simulink library "NeuroModelerLibrary"  (Simulink 10.2)
settings: Solver=ode45  StartTime=0.0  StopTime=10.0  RelTol=1e-3
libraries: $bdroot x672, simulink x5, neural x2
(part 5 of 5)

== system NeuroModelerLibrary/Simple Cells/Simple Cell - Inertial/Synapse ==
  In1 : Inport
  Constant1 : Constant  Value=0
  Constant4 : Constant  Value=DecompositionTC
  Constant5 : Constant  Value=SecretionTC
  Fcn : Fcn  Expr=u*u*ksi
  Gain : Gain  Gain=1/gamma  SaturateOnIntegerOverflow=on  OutDataTypeStr=Inherit: Same as input  ParamDataTypeStr=Inherit: Same as input
  Gain1 : Gain  SaturateOnIntegerOverflow=on  OutDataTypeStr=Inherit: Same as input  ParamDataTypeStr=Inherit: Same as input
  Inertial Link : $bdroot/Support/Inertial Link
  Sum : Sum  Inputs=+-  SaturateOnIntegerOverflow=on
  Switch1 : Switch
  Switch2 : Switch  Threshold=1
  Out1 : Outport  VectorParamsAs1DForOutWhenUnconnected=off
  wires:
  Switch1/1 -> Out1/1
  Gain1/1 -> Inertial Link/1
  Constant1/1 -> Switch1/3
  Gain/1 -> Switch1/1, Switch1/2
  Switch2/1 -> Inertial Link/2
  Constant5/1 -> Switch2/1
  Constant4/1 -> Switch2/3
  Inertial Link/1 -> Sum/1
  Sum/1 -> Gain/1
  In1/1 -> Gain1/1, Switch2/2
  Fcn/1 -> Sum/2

== system NeuroModelerLibrary/Simple Cells/Simple Cell - Inertial/Synapse1 ==
  In1 : Inport
  Constant1 : Constant  Value=0
  Constant4 : Constant  Value=DecompositionTC
  Constant5 : Constant  Value=SecretionTC
  Fcn : Fcn  Expr=u*u*ksi
  Gain : Gain  Gain=1/gamma  SaturateOnIntegerOverflow=on  OutDataTypeStr=Inherit: Same as input  ParamDataTypeStr=Inherit: Same as input
  Gain1 : Gain  SaturateOnIntegerOverflow=on  OutDataTypeStr=Inherit: Same as input  ParamDataTypeStr=Inherit: Same as input
  Inertial Link : $bdroot/Support/Inertial Link
  Sum : Sum  Inputs=+-  SaturateOnIntegerOverflow=on
  Switch1 : Switch
  Switch2 : Switch  Threshold=1
  Out1 : Outport  VectorParamsAs1DForOutWhenUnconnected=off
  wires:
  Switch1/1 -> Out1/1
  Gain1/1 -> Inertial Link/1
  Constant1/1 -> Switch1/3
  Gain/1 -> Switch1/1, Switch1/2
  Switch2/1 -> Inertial Link/2
  Constant5/1 -> Switch2/1
  Constant4/1 -> Switch2/3
  Inertial Link/1 -> Sum/1, Fcn/1
  Sum/1 -> Gain/1
  In1/1 -> Gain1/1, Switch2/2

== system NeuroModelerLibrary/Simple Cells/Simple Cell MembraneCap/Synapse ==
  In1 : Inport
  Constant1 : Constant  Value=0
  Constant4 : Constant  Value=DecompositionTC
  Constant5 : Constant  Value=SecretionTC
  Fcn : Fcn  Expr=u*u*ksi
  Gain : Gain  Gain=1/gamma  SaturateOnIntegerOverflow=on  OutDataTypeStr=Inherit: Same as input  ParamDataTypeStr=Inherit: Same as input
  Gain1 : Gain  SaturateOnIntegerOverflow=on  OutDataTypeStr=Inherit: Same as input  ParamDataTypeStr=Inherit: Same as input
  Inertial Link : $bdroot/Support/Inertial Link  SystemSampleTime=-1  VariantActivationTime=update diagram  Latency=0  AutoFrameSizeCalculation=off
  Sum : Sum  Inputs=+-  SaturateOnIntegerOverflow=on
  Switch1 : Switch
  Switch2 : Switch  Threshold=1
  Out1 : Outport
  wires:
  Fcn/1 -> Sum/2
  In1/1 -> Switch2/2, Gain1/1
  Sum/1 -> Gain/1
  Inertial Link/1 -> Sum/1
  Constant4/1 -> Switch2/3
  Constant5/1 -> Switch2/1
  Switch2/1 -> Inertial Link/2
  Gain/1 -> Switch1/2, Switch1/1
  Constant1/1 -> Switch1/3
  Gain1/1 -> Inertial Link/1
  Switch1/1 -> Out1/1

== system NeuroModelerLibrary/Simple Cells/Simple Cell MembraneCap/Synapse1 ==
  In1 : Inport
  Constant1 : Constant  Value=0
  Constant4 : Constant  Value=DecompositionTC
  Constant5 : Constant  Value=SecretionTC
  Fcn : Fcn  Expr=u*u*ksi
  Gain : Gain  Gain=1/gamma  SaturateOnIntegerOverflow=on  OutDataTypeStr=Inherit: Same as input  ParamDataTypeStr=Inherit: Same as input
  Gain1 : Gain  SaturateOnIntegerOverflow=on  OutDataTypeStr=Inherit: Same as input  ParamDataTypeStr=Inherit: Same as input
  Inertial Link : $bdroot/Support/Inertial Link  SystemSampleTime=-1  VariantActivationTime=update diagram  Latency=0  AutoFrameSizeCalculation=off
  Sum : Sum  Inputs=+-  SaturateOnIntegerOverflow=on
  Switch1 : Switch
  Switch2 : Switch  Threshold=1
  Out1 : Outport
  wires:
  In1/1 -> Switch2/2, Gain1/1
  Sum/1 -> Gain/1
  Inertial Link/1 -> Fcn/1, Sum/1
  Constant4/1 -> Switch2/3
  Constant5/1 -> Switch2/1
  Switch2/1 -> Inertial Link/2
  Gain/1 -> Switch1/2, Switch1/1
  Constant1/1 -> Switch1/3
  Gain1/1 -> Inertial Link/1
  Switch1/1 -> Out1/1

== system NeuroModelerLibrary/Simple Cells/Simple Cell MembraneCap[2]/Synapse ==
  In1 : Inport
  Constant1 : Constant  Value=0
  Constant4 : Constant  Value=DecompositionTC
  Constant5 : Constant  Value=SecretionTC
  Fcn : Fcn  Expr=u*u*ksi
  Gain : Gain  Gain=1/gamma  SaturateOnIntegerOverflow=on  OutDataTypeStr=Inherit: Same as input  ParamDataTypeStr=Inherit: Same as input
  Gain1 : Gain  SaturateOnIntegerOverflow=on  OutDataTypeStr=Inherit: Same as input  ParamDataTypeStr=Inherit: Same as input
  Inertial Link : $bdroot/Support/Inertial Link  SystemSampleTime=-1  VariantActivationTime=update diagram  Latency=0  AutoFrameSizeCalculation=off
  Sum : Sum  Inputs=+-  SaturateOnIntegerOverflow=on
  Switch1 : Switch
  Switch2 : Switch  Threshold=1
  Out1 : Outport
  wires:
  Fcn/1 -> Sum/2
  In1/1 -> Switch2/2, Gain1/1
  Sum/1 -> Gain/1
  Inertial Link/1 -> Sum/1
  Constant4/1 -> Switch2/3
  Constant5/1 -> Switch2/1
  Switch2/1 -> Inertial Link/2
  Gain/1 -> Switch1/2, Switch1/1
  Constant1/1 -> Switch1/3
  Gain1/1 -> Inertial Link/1
  Switch1/1 -> Out1/1

== system NeuroModelerLibrary/Simple Cells/Simple Cell MembraneCap[2]/Synapse1 ==
  In1 : Inport
  Constant1 : Constant  Value=0
  Constant4 : Constant  Value=DecompositionTC
  Constant5 : Constant  Value=SecretionTC
  Fcn : Fcn  Expr=u*u*ksi
  Gain : Gain  Gain=1/gamma  SaturateOnIntegerOverflow=on  OutDataTypeStr=Inherit: Same as input  ParamDataTypeStr=Inherit: Same as input
  Gain1 : Gain  SaturateOnIntegerOverflow=on  OutDataTypeStr=Inherit: Same as input  ParamDataTypeStr=Inherit: Same as input
  Inertial Link : $bdroot/Support/Inertial Link  SystemSampleTime=-1  VariantActivationTime=update diagram  Latency=0  AutoFrameSizeCalculation=off
  Sum : Sum  Inputs=+-  SaturateOnIntegerOverflow=on
  Switch1 : Switch
  Switch2 : Switch  Threshold=1
  Out1 : Outport
  wires:
  In1/1 -> Switch2/2, Gain1/1
  Sum/1 -> Gain/1
  Inertial Link/1 -> Fcn/1, Sum/1
  Constant4/1 -> Switch2/3
  Constant5/1 -> Switch2/1
  Switch2/1 -> Inertial Link/2
  Gain/1 -> Switch1/2, Switch1/1
  Constant1/1 -> Switch1/3
  Gain1/1 -> Inertial Link/1
  Switch1/1 -> Out1/1

== system NeuroModelerLibrary/Sized Cells/Cell IaF 1x4/IaF LTZone6 ==
  Potential : Inport
  Constant2 : Constant
  Constant6 : Constant  Value=0
  S1 : Switch  Threshold=V_th  SaturateOnIntegerOverflow=on  InputSameDT=on
  Out : Outport
  Out Potential : Outport  Port=2
  wires:
  Constant2/1 -> S1/1
  Constant6/1 -> S1/3
  Potential/1 -> Out Potential/1, S1/2
  S1/1 -> Out/1

== system NeuroModelerLibrary/Sized Cells/Cell IaF 1x4/IaF Membrane Segment18 ==
  Synapses : Inport
  Resting Potential : Inport  Port=2
  Reset Signal : Inport  Port=3
  Constant1 : Constant  Value=V_reset
  Constant10 : Constant  Value=tau_m
  Constant12 : Constant  Value=I_const
  Gain3 : Gain  Gain=tau_m/Cm
  Inertial Link With Reset1 : $bdroot/Support/Inertial Link With Reset  SystemSampleTime=-1  VariantActivationTime=update diagram  Latency=0  AutoFrameSizeCalculation=off
  Sum1 : Sum
  Sum3 : Sum
  Out1 : Outport
  wires:
  Resting Potential/1 -> Sum3/2
  Constant10/1 -> Inertial Link With Reset1/2
  Synapses/1 -> Sum1/1
  Sum1/1 -> Gain3/1
  Constant12/1 -> Sum1/2
  Sum3/1 -> Inertial Link With Reset1/1  "Value"
  Inertial Link With Reset1/1 -> Out1/1
  Constant1/1 -> Inertial Link With Reset1/3
  Gain3/1 -> Sum3/1  "Input"
  Reset Signal/1 -> Inertial Link With Reset1/4

== system NeuroModelerLibrary/Sized Cells/Cell IaF 1x4/IaF Membrane Segment19 ==
  Synapses : Inport
  Resting Potential : Inport  Port=2
  Reset Signal : Inport  Port=3
  Constant1 : Constant  Value=V_reset
  Constant10 : Constant  Value=tau_m
  Constant12 : Constant  Value=I_const
  Gain3 : Gain  Gain=tau_m/Cm
  Inertial Link With Reset1 : $bdroot/Support/Inertial Link With Reset  SystemSampleTime=-1  VariantActivationTime=update diagram  Latency=0  AutoFrameSizeCalculation=off
  Sum1 : Sum
  Sum3 : Sum
  Out1 : Outport
  wires:
  Resting Potential/1 -> Sum3/2
  Constant10/1 -> Inertial Link With Reset1/2
  Synapses/1 -> Sum1/1
  Sum1/1 -> Gain3/1
  Constant12/1 -> Sum1/2
  Sum3/1 -> Inertial Link With Reset1/1  "Value"
  Inertial Link With Reset1/1 -> Out1/1
  Constant1/1 -> Inertial Link With Reset1/3
  Gain3/1 -> Sum3/1  "Input"
  Reset Signal/1 -> Inertial Link With Reset1/4

== system NeuroModelerLibrary/Sized Cells/Cell IaF 1x4/IaF Membrane Segment20 ==
  Synapses : Inport
  Resting Potential : Inport  Port=2
  Reset Signal : Inport  Port=3
  Constant1 : Constant  Value=V_reset
  Constant10 : Constant  Value=tau_m
  Constant12 : Constant  Value=I_const
  Gain3 : Gain  Gain=tau_m/Cm
  Inertial Link With Reset1 : $bdroot/Support/Inertial Link With Reset  SystemSampleTime=-1  VariantActivationTime=update diagram  Latency=0  AutoFrameSizeCalculation=off
  Sum1 : Sum
  Sum3 : Sum
  Out1 : Outport
  wires:
  Resting Potential/1 -> Sum3/2
  Constant10/1 -> Inertial Link With Reset1/2
  Synapses/1 -> Sum1/1
  Sum1/1 -> Gain3/1
  Constant12/1 -> Sum1/2
  Sum3/1 -> Inertial Link With Reset1/1  "Value"
  Inertial Link With Reset1/1 -> Out1/1
  Constant1/1 -> Inertial Link With Reset1/3
  Gain3/1 -> Sum3/1  "Input"
  Reset Signal/1 -> Inertial Link With Reset1/4

== system NeuroModelerLibrary/Sized Cells/Cell IaF 1x4/IaF Membrane Segment21 ==
  Synapses : Inport
  Resting Potential : Inport  Port=2
  Reset Signal : Inport  Port=3
  Constant1 : Constant  Value=V_reset
  Constant10 : Constant  Value=tau_m
  Constant12 : Constant  Value=I_const
  Gain3 : Gain  Gain=tau_m/Cm
  Inertial Link With Reset1 : $bdroot/Support/Inertial Link With Reset  SystemSampleTime=-1  VariantActivationTime=update diagram  Latency=0  AutoFrameSizeCalculation=off
  Sum1 : Sum
  Sum3 : Sum
  Out1 : Outport
  wires:
  Resting Potential/1 -> Sum3/2
  Constant10/1 -> Inertial Link With Reset1/2
  Synapses/1 -> Sum1/1
  Sum1/1 -> Gain3/1
  Constant12/1 -> Sum1/2
  Sum3/1 -> Inertial Link With Reset1/1  "Value"
  Inertial Link With Reset1/1 -> Out1/1
  Constant1/1 -> Inertial Link With Reset1/3
  Gain3/1 -> Sum3/1  "Input"
  Reset Signal/1 -> Inertial Link With Reset1/4

== system NeuroModelerLibrary/Sized Cells/Cell IaF 1x4-Syn4/IaF LTZone1 ==
  Potential : Inport
  Constant2 : Constant
  Constant6 : Constant  Value=0
  S1 : Switch  Threshold=V_th  SaturateOnIntegerOverflow=on  InputSameDT=on
  Out : Outport
  Out Potential : Outport  Port=2
  wires:
  Constant2/1 -> S1/1
  Constant6/1 -> S1/3
  Potential/1 -> Out Potential/1, S1/2
  S1/1 -> Out/1

== system NeuroModelerLibrary/Sized Cells/Cell IaF 1x4-Syn4/IaF Membrane Segment1 ==
  Synapses : Inport
  Resting Potential : Inport  Port=2
  Reset Signal : Inport  Port=3
  Constant1 : Constant  Value=V_reset
  Constant10 : Constant  Value=tau_m
  Constant12 : Constant  Value=I_const
  Gain3 : Gain  Gain=tau_m/Cm
  Inertial Link With Reset1 : $bdroot/Support/Inertial Link With Reset  SystemSampleTime=-1  VariantActivationTime=update diagram  Latency=0  AutoFrameSizeCalculation=off
  Sum1 : Sum
  Sum3 : Sum
  Out1 : Outport
  wires:
  Resting Potential/1 -> Sum3/2
  Constant10/1 -> Inertial Link With Reset1/2
  Synapses/1 -> Sum1/1
  Sum1/1 -> Gain3/1
  Constant12/1 -> Sum1/2
  Sum3/1 -> Inertial Link With Reset1/1  "Value"
  Inertial Link With Reset1/1 -> Out1/1
  Constant1/1 -> Inertial Link With Reset1/3
  Gain3/1 -> Sum3/1  "Input"
  Reset Signal/1 -> Inertial Link With Reset1/4

== system NeuroModelerLibrary/Sized Cells/Cell IaF 1x4-Syn4/IaF Membrane Segment2 ==
  Synapses : Inport
  Resting Potential : Inport  Port=2
  Reset Signal : Inport  Port=3
  Constant1 : Constant  Value=V_reset
  Constant10 : Constant  Value=tau_m
  Constant12 : Constant  Value=I_const
  Gain3 : Gain  Gain=tau_m/Cm
  Inertial Link With Reset1 : $bdroot/Support/Inertial Link With Reset  SystemSampleTime=-1  VariantActivationTime=update diagram  Latency=0  AutoFrameSizeCalculation=off
  Sum1 : Sum
  Sum3 : Sum
  Out1 : Outport
  wires:
  Resting Potential/1 -> Sum3/2
  Constant10/1 -> Inertial Link With Reset1/2
  Synapses/1 -> Sum1/1
  Sum1/1 -> Gain3/1
  Constant12/1 -> Sum1/2
  Sum3/1 -> Inertial Link With Reset1/1  "Value"
  Inertial Link With Reset1/1 -> Out1/1
  Constant1/1 -> Inertial Link With Reset1/3
  Gain3/1 -> Sum3/1  "Input"
  Reset Signal/1 -> Inertial Link With Reset1/4

== system NeuroModelerLibrary/Sized Cells/Cell IaF 1x4-Syn4/IaF Membrane Segment3 ==
  Synapses : Inport
  Resting Potential : Inport  Port=2
  Reset Signal : Inport  Port=3
  Constant1 : Constant  Value=V_reset
  Constant10 : Constant  Value=tau_m
  Constant12 : Constant  Value=I_const
  Gain3 : Gain  Gain=tau_m/Cm
  Inertial Link With Reset1 : $bdroot/Support/Inertial Link With Reset  SystemSampleTime=-1  VariantActivationTime=update diagram  Latency=0  AutoFrameSizeCalculation=off
  Sum1 : Sum
  Sum3 : Sum
  Out1 : Outport
  wires:
  Resting Potential/1 -> Sum3/2
  Constant10/1 -> Inertial Link With Reset1/2
  Synapses/1 -> Sum1/1
  Sum1/1 -> Gain3/1
  Constant12/1 -> Sum1/2
  Sum3/1 -> Inertial Link With Reset1/1  "Value"
  Inertial Link With Reset1/1 -> Out1/1
  Constant1/1 -> Inertial Link With Reset1/3
  Gain3/1 -> Sum3/1  "Input"
  Reset Signal/1 -> Inertial Link With Reset1/4

== system NeuroModelerLibrary/Sized Cells/Cell IaF 1x4-Syn4/IaF Membrane Segment4 ==
  Synapses : Inport
  Resting Potential : Inport  Port=2
  Reset Signal : Inport  Port=3
  Constant1 : Constant  Value=V_reset
  Constant10 : Constant  Value=tau_m
  Constant12 : Constant  Value=I_const
  Gain3 : Gain  Gain=tau_m/Cm
  Inertial Link With Reset1 : $bdroot/Support/Inertial Link With Reset  SystemSampleTime=-1  VariantActivationTime=update diagram  Latency=0  AutoFrameSizeCalculation=off
  Sum1 : Sum
  Sum3 : Sum
  Out1 : Outport
  wires:
  Resting Potential/1 -> Sum3/2
  Constant10/1 -> Inertial Link With Reset1/2
  Synapses/1 -> Sum1/1
  Sum1/1 -> Gain3/1
  Constant12/1 -> Sum1/2
  Sum3/1 -> Inertial Link With Reset1/1  "Value"
  Inertial Link With Reset1/1 -> Out1/1
  Constant1/1 -> Inertial Link With Reset1/3
  Gain3/1 -> Sum3/1  "Input"
  Reset Signal/1 -> Inertial Link With Reset1/4

== system NeuroModelerLibrary/Sized Cells/Cell IaF 2x4/IaF LTZone7 ==
  Potential : Inport
  Constant2 : Constant
  Constant6 : Constant  Value=0
  S1 : Switch  Threshold=V_th  SaturateOnIntegerOverflow=on  InputSameDT=on
  Out : Outport
  Out Potential : Outport  Port=2
  wires:
  Constant2/1 -> S1/1
  Constant6/1 -> S1/3
  Potential/1 -> Out Potential/1, S1/2
  S1/1 -> Out/1

== system NeuroModelerLibrary/Sized Cells/Cell IaF 2x4/IaF Membrane Segment22 ==
  Synapses : Inport
  Resting Potential : Inport  Port=2
  Reset Signal : Inport  Port=3
  Constant1 : Constant  Value=V_reset
  Constant10 : Constant  Value=tau_m
  Constant12 : Constant  Value=I_const
  Gain3 : Gain  Gain=tau_m/Cm
  Inertial Link With Reset1 : $bdroot/Support/Inertial Link With Reset  SystemSampleTime=-1  VariantActivationTime=update diagram  Latency=0  AutoFrameSizeCalculation=off
  Sum1 : Sum
  Sum3 : Sum
  Out1 : Outport
  wires:
  Resting Potential/1 -> Sum3/2
  Constant10/1 -> Inertial Link With Reset1/2
  Synapses/1 -> Sum1/1
  Sum1/1 -> Gain3/1
  Constant12/1 -> Sum1/2
  Sum3/1 -> Inertial Link With Reset1/1  "Value"
  Inertial Link With Reset1/1 -> Out1/1
  Constant1/1 -> Inertial Link With Reset1/3
  Gain3/1 -> Sum3/1  "Input"
  Reset Signal/1 -> Inertial Link With Reset1/4

== system NeuroModelerLibrary/Sized Cells/Cell IaF 2x4/IaF Membrane Segment23 ==
  Synapses : Inport
  Resting Potential : Inport  Port=2
  Reset Signal : Inport  Port=3
  Constant1 : Constant  Value=V_reset
  Constant10 : Constant  Value=tau_m
  Constant12 : Constant  Value=I_const
  Gain3 : Gain  Gain=tau_m/Cm
  Inertial Link With Reset1 : $bdroot/Support/Inertial Link With Reset  SystemSampleTime=-1  VariantActivationTime=update diagram  Latency=0  AutoFrameSizeCalculation=off
  Sum1 : Sum
  Sum3 : Sum
  Out1 : Outport
  wires:
  Resting Potential/1 -> Sum3/2
  Constant10/1 -> Inertial Link With Reset1/2
  Synapses/1 -> Sum1/1
  Sum1/1 -> Gain3/1
  Constant12/1 -> Sum1/2
  Sum3/1 -> Inertial Link With Reset1/1  "Value"
  Inertial Link With Reset1/1 -> Out1/1
  Constant1/1 -> Inertial Link With Reset1/3
  Gain3/1 -> Sum3/1  "Input"
  Reset Signal/1 -> Inertial Link With Reset1/4

== system NeuroModelerLibrary/Sized Cells/Cell IaF 2x4/IaF Membrane Segment24 ==
  Synapses : Inport
  Resting Potential : Inport  Port=2
  Reset Signal : Inport  Port=3
  Constant1 : Constant  Value=V_reset
  Constant10 : Constant  Value=tau_m
  Constant12 : Constant  Value=I_const
  Gain3 : Gain  Gain=tau_m/Cm
  Inertial Link With Reset1 : $bdroot/Support/Inertial Link With Reset  SystemSampleTime=-1  VariantActivationTime=update diagram  Latency=0  AutoFrameSizeCalculation=off
  Sum1 : Sum
  Sum3 : Sum
  Out1 : Outport
  wires:
  Resting Potential/1 -> Sum3/2
  Constant10/1 -> Inertial Link With Reset1/2
  Synapses/1 -> Sum1/1
  Sum1/1 -> Gain3/1
  Constant12/1 -> Sum1/2
  Sum3/1 -> Inertial Link With Reset1/1  "Value"
  Inertial Link With Reset1/1 -> Out1/1
  Constant1/1 -> Inertial Link With Reset1/3
  Gain3/1 -> Sum3/1  "Input"
  Reset Signal/1 -> Inertial Link With Reset1/4

== system NeuroModelerLibrary/Sized Cells/Cell IaF 2x4/IaF Membrane Segment25 ==
  Synapses : Inport
  Resting Potential : Inport  Port=2
  Reset Signal : Inport  Port=3
  Constant1 : Constant  Value=V_reset
  Constant10 : Constant  Value=tau_m
  Constant12 : Constant  Value=I_const
  Gain3 : Gain  Gain=tau_m/Cm
  Inertial Link With Reset1 : $bdroot/Support/Inertial Link With Reset  SystemSampleTime=-1  VariantActivationTime=update diagram  Latency=0  AutoFrameSizeCalculation=off
  Sum1 : Sum
  Sum3 : Sum
  Out1 : Outport
  wires:
  Resting Potential/1 -> Sum3/2
  Constant10/1 -> Inertial Link With Reset1/2
  Synapses/1 -> Sum1/1
  Sum1/1 -> Gain3/1
  Constant12/1 -> Sum1/2
  Sum3/1 -> Inertial Link With Reset1/1  "Value"
  Inertial Link With Reset1/1 -> Out1/1
  Constant1/1 -> Inertial Link With Reset1/3
  Gain3/1 -> Sum3/1  "Input"
  Reset Signal/1 -> Inertial Link With Reset1/4

== system NeuroModelerLibrary/Sized Cells/Cell IaF 2x4/IaF Membrane Segment26 ==
  Synapses : Inport
  Resting Potential : Inport  Port=2
  Reset Signal : Inport  Port=3
  Constant1 : Constant  Value=V_reset
  Constant10 : Constant  Value=tau_m
  Constant12 : Constant  Value=I_const
  Gain3 : Gain  Gain=tau_m/Cm
  Inertial Link With Reset1 : $bdroot/Support/Inertial Link With Reset  SystemSampleTime=-1  VariantActivationTime=update diagram  Latency=0  AutoFrameSizeCalculation=off
  Sum1 : Sum
  Sum3 : Sum
  Out1 : Outport
  wires:
  Resting Potential/1 -> Sum3/2
  Constant10/1 -> Inertial Link With Reset1/2
  Synapses/1 -> Sum1/1
  Sum1/1 -> Gain3/1
  Constant12/1 -> Sum1/2
  Sum3/1 -> Inertial Link With Reset1/1  "Value"
  Inertial Link With Reset1/1 -> Out1/1
  Constant1/1 -> Inertial Link With Reset1/3
  Gain3/1 -> Sum3/1  "Input"
  Reset Signal/1 -> Inertial Link With Reset1/4

== system NeuroModelerLibrary/Sized Cells/Cell IaF 3x4/IaF LTZone8 ==
  Potential : Inport
  Constant2 : Constant
  Constant6 : Constant  Value=0
  S1 : Switch  Threshold=V_th  SaturateOnIntegerOverflow=on  InputSameDT=on
  Out : Outport
  Out Potential : Outport  Port=2
  wires:
  Constant2/1 -> S1/1
  Constant6/1 -> S1/3
  Potential/1 -> Out Potential/1, S1/2
  S1/1 -> Out/1

== system NeuroModelerLibrary/Sized Cells/Cell IaF 3x4/IaF Membrane Segment27 ==
  Synapses : Inport
  Resting Potential : Inport  Port=2
  Reset Signal : Inport  Port=3
  Constant1 : Constant  Value=V_reset
  Constant10 : Constant  Value=tau_m
  Constant12 : Constant  Value=I_const
  Gain3 : Gain  Gain=tau_m/Cm
  Inertial Link With Reset1 : $bdroot/Support/Inertial Link With Reset  SystemSampleTime=-1  VariantActivationTime=update diagram  Latency=0  AutoFrameSizeCalculation=off
  Sum1 : Sum
  Sum3 : Sum
  Out1 : Outport
  wires:
  Resting Potential/1 -> Sum3/2
  Constant10/1 -> Inertial Link With Reset1/2
  Synapses/1 -> Sum1/1
  Sum1/1 -> Gain3/1
  Constant12/1 -> Sum1/2
  Sum3/1 -> Inertial Link With Reset1/1  "Value"
  Inertial Link With Reset1/1 -> Out1/1
  Constant1/1 -> Inertial Link With Reset1/3
  Gain3/1 -> Sum3/1  "Input"
  Reset Signal/1 -> Inertial Link With Reset1/4

== system NeuroModelerLibrary/Sized Cells/Cell IaF 3x4/IaF Membrane Segment28 ==
  Synapses : Inport
  Resting Potential : Inport  Port=2
  Reset Signal : Inport  Port=3
  Constant1 : Constant  Value=V_reset
  Constant10 : Constant  Value=tau_m
  Constant12 : Constant  Value=I_const
  Gain3 : Gain  Gain=tau_m/Cm
  Inertial Link With Reset1 : $bdroot/Support/Inertial Link With Reset  SystemSampleTime=-1  VariantActivationTime=update diagram  Latency=0  AutoFrameSizeCalculation=off
  Sum1 : Sum
  Sum3 : Sum
  Out1 : Outport
  wires:
  Resting Potential/1 -> Sum3/2
  Constant10/1 -> Inertial Link With Reset1/2
  Synapses/1 -> Sum1/1
  Sum1/1 -> Gain3/1
  Constant12/1 -> Sum1/2
  Sum3/1 -> Inertial Link With Reset1/1  "Value"
  Inertial Link With Reset1/1 -> Out1/1
  Constant1/1 -> Inertial Link With Reset1/3
  Gain3/1 -> Sum3/1  "Input"
  Reset Signal/1 -> Inertial Link With Reset1/4

== system NeuroModelerLibrary/Sized Cells/Cell IaF 3x4/IaF Membrane Segment29 ==
  Synapses : Inport
  Resting Potential : Inport  Port=2
  Reset Signal : Inport  Port=3
  Constant1 : Constant  Value=V_reset
  Constant10 : Constant  Value=tau_m
  Constant12 : Constant  Value=I_const
  Gain3 : Gain  Gain=tau_m/Cm
  Inertial Link With Reset1 : $bdroot/Support/Inertial Link With Reset  SystemSampleTime=-1  VariantActivationTime=update diagram  Latency=0  AutoFrameSizeCalculation=off
  Sum1 : Sum
  Sum3 : Sum
  Out1 : Outport
  wires:
  Resting Potential/1 -> Sum3/2
  Constant10/1 -> Inertial Link With Reset1/2
  Synapses/1 -> Sum1/1
  Sum1/1 -> Gain3/1
  Constant12/1 -> Sum1/2
  Sum3/1 -> Inertial Link With Reset1/1  "Value"
  Inertial Link With Reset1/1 -> Out1/1
  Constant1/1 -> Inertial Link With Reset1/3
  Gain3/1 -> Sum3/1  "Input"
  Reset Signal/1 -> Inertial Link With Reset1/4

== system NeuroModelerLibrary/Sized Cells/Cell IaF 3x4/IaF Membrane Segment30 ==
  Synapses : Inport
  Resting Potential : Inport  Port=2
  Reset Signal : Inport  Port=3
  Constant1 : Constant  Value=V_reset
  Constant10 : Constant  Value=tau_m
  Constant12 : Constant  Value=I_const
  Gain3 : Gain  Gain=tau_m/Cm
  Inertial Link With Reset1 : $bdroot/Support/Inertial Link With Reset  SystemSampleTime=-1  VariantActivationTime=update diagram  Latency=0  AutoFrameSizeCalculation=off
  Sum1 : Sum
  Sum3 : Sum
  Out1 : Outport
  wires:
  Resting Potential/1 -> Sum3/2
  Constant10/1 -> Inertial Link With Reset1/2
  Synapses/1 -> Sum1/1
  Sum1/1 -> Gain3/1
  Constant12/1 -> Sum1/2
  Sum3/1 -> Inertial Link With Reset1/1  "Value"
  Inertial Link With Reset1/1 -> Out1/1
  Constant1/1 -> Inertial Link With Reset1/3
  Gain3/1 -> Sum3/1  "Input"
  Reset Signal/1 -> Inertial Link With Reset1/4

== system NeuroModelerLibrary/Sized Cells/Cell IaF 3x4/IaF Membrane Segment31 ==
  Synapses : Inport
  Resting Potential : Inport  Port=2
  Reset Signal : Inport  Port=3
  Constant1 : Constant  Value=V_reset
  Constant10 : Constant  Value=tau_m
  Constant12 : Constant  Value=I_const
  Gain3 : Gain  Gain=tau_m/Cm
  Inertial Link With Reset1 : $bdroot/Support/Inertial Link With Reset  SystemSampleTime=-1  VariantActivationTime=update diagram  Latency=0  AutoFrameSizeCalculation=off
  Sum1 : Sum
  Sum3 : Sum
  Out1 : Outport
  wires:
  Resting Potential/1 -> Sum3/2
  Constant10/1 -> Inertial Link With Reset1/2
  Synapses/1 -> Sum1/1
  Sum1/1 -> Gain3/1
  Constant12/1 -> Sum1/2
  Sum3/1 -> Inertial Link With Reset1/1  "Value"
  Inertial Link With Reset1/1 -> Out1/1
  Constant1/1 -> Inertial Link With Reset1/3
  Gain3/1 -> Sum3/1  "Input"
  Reset Signal/1 -> Inertial Link With Reset1/4

== system NeuroModelerLibrary/Sized Cells/Cell IaF 3x4/IaF Membrane Segment32 ==
  Synapses : Inport
  Resting Potential : Inport  Port=2
  Reset Signal : Inport  Port=3
  Constant1 : Constant  Value=V_reset
  Constant10 : Constant  Value=tau_m
  Constant12 : Constant  Value=I_const
  Gain3 : Gain  Gain=tau_m/Cm
  Inertial Link With Reset1 : $bdroot/Support/Inertial Link With Reset  SystemSampleTime=-1  VariantActivationTime=update diagram  Latency=0  AutoFrameSizeCalculation=off
  Sum1 : Sum
  Sum3 : Sum
  Out1 : Outport
  wires:
  Resting Potential/1 -> Sum3/2
  Constant10/1 -> Inertial Link With Reset1/2
  Synapses/1 -> Sum1/1
  Sum1/1 -> Gain3/1
  Constant12/1 -> Sum1/2
  Sum3/1 -> Inertial Link With Reset1/1  "Value"
  Inertial Link With Reset1/1 -> Out1/1
  Constant1/1 -> Inertial Link With Reset1/3
  Gain3/1 -> Sum3/1  "Input"
  Reset Signal/1 -> Inertial Link With Reset1/4

== system NeuroModelerLibrary/Sized Cells/Cell IaF 4x4/IaF LTZone9 ==
  Potential : Inport
  Constant2 : Constant
  Constant6 : Constant  Value=0
  S1 : Switch  Threshold=V_th  SaturateOnIntegerOverflow=on  InputSameDT=on
  Out : Outport
  Out Potential : Outport  Port=2
  wires:
  Constant2/1 -> S1/1
  Constant6/1 -> S1/3
  Potential/1 -> Out Potential/1, S1/2
  S1/1 -> Out/1

== system NeuroModelerLibrary/Sized Cells/Cell IaF 4x4/IaF Membrane Segment33 ==
  Synapses : Inport
  Resting Potential : Inport  Port=2
  Reset Signal : Inport  Port=3
  Constant1 : Constant  Value=V_reset
  Constant10 : Constant  Value=tau_m
  Constant12 : Constant  Value=I_const
  Gain3 : Gain  Gain=tau_m/Cm
  Inertial Link With Reset1 : $bdroot/Support/Inertial Link With Reset  SystemSampleTime=-1  VariantActivationTime=update diagram  Latency=0  AutoFrameSizeCalculation=off
  Sum1 : Sum
  Sum3 : Sum
  Out1 : Outport
  wires:
  Resting Potential/1 -> Sum3/2
  Constant10/1 -> Inertial Link With Reset1/2
  Synapses/1 -> Sum1/1
  Sum1/1 -> Gain3/1
  Constant12/1 -> Sum1/2
  Sum3/1 -> Inertial Link With Reset1/1  "Value"
  Inertial Link With Reset1/1 -> Out1/1
  Constant1/1 -> Inertial Link With Reset1/3
  Gain3/1 -> Sum3/1  "Input"
  Reset Signal/1 -> Inertial Link With Reset1/4

== system NeuroModelerLibrary/Sized Cells/Cell IaF 4x4/IaF Membrane Segment34 ==
  Synapses : Inport
  Resting Potential : Inport  Port=2
  Reset Signal : Inport  Port=3
  Constant1 : Constant  Value=V_reset
  Constant10 : Constant  Value=tau_m
  Constant12 : Constant  Value=I_const
  Gain3 : Gain  Gain=tau_m/Cm
  Inertial Link With Reset1 : $bdroot/Support/Inertial Link With Reset  SystemSampleTime=-1  VariantActivationTime=update diagram  Latency=0  AutoFrameSizeCalculation=off
  Sum1 : Sum
  Sum3 : Sum
  Out1 : Outport
  wires:
  Resting Potential/1 -> Sum3/2
  Constant10/1 -> Inertial Link With Reset1/2
  Synapses/1 -> Sum1/1
  Sum1/1 -> Gain3/1
  Constant12/1 -> Sum1/2
  Sum3/1 -> Inertial Link With Reset1/1  "Value"
  Inertial Link With Reset1/1 -> Out1/1
  Constant1/1 -> Inertial Link With Reset1/3
  Gain3/1 -> Sum3/1  "Input"
  Reset Signal/1 -> Inertial Link With Reset1/4

== system NeuroModelerLibrary/Sized Cells/Cell IaF 4x4/IaF Membrane Segment35 ==
  Synapses : Inport
  Resting Potential : Inport  Port=2
  Reset Signal : Inport  Port=3
  Constant1 : Constant  Value=V_reset
  Constant10 : Constant  Value=tau_m
  Constant12 : Constant  Value=I_const
  Gain3 : Gain  Gain=tau_m/Cm
  Inertial Link With Reset1 : $bdroot/Support/Inertial Link With Reset  SystemSampleTime=-1  VariantActivationTime=update diagram  Latency=0  AutoFrameSizeCalculation=off
  Sum1 : Sum
  Sum3 : Sum
  Out1 : Outport
  wires:
  Resting Potential/1 -> Sum3/2
  Constant10/1 -> Inertial Link With Reset1/2
  Synapses/1 -> Sum1/1
  Sum1/1 -> Gain3/1
  Constant12/1 -> Sum1/2
  Sum3/1 -> Inertial Link With Reset1/1  "Value"
  Inertial Link With Reset1/1 -> Out1/1
  Constant1/1 -> Inertial Link With Reset1/3
  Gain3/1 -> Sum3/1  "Input"
  Reset Signal/1 -> Inertial Link With Reset1/4

== system NeuroModelerLibrary/Sized Cells/Cell IaF 4x4/IaF Membrane Segment36 ==
  Synapses : Inport
  Resting Potential : Inport  Port=2
  Reset Signal : Inport  Port=3
  Constant1 : Constant  Value=V_reset
  Constant10 : Constant  Value=tau_m
  Constant12 : Constant  Value=I_const
  Gain3 : Gain  Gain=tau_m/Cm
  Inertial Link With Reset1 : $bdroot/Support/Inertial Link With Reset  SystemSampleTime=-1  VariantActivationTime=update diagram  Latency=0  AutoFrameSizeCalculation=off
  Sum1 : Sum
  Sum3 : Sum
  Out1 : Outport
  wires:
  Resting Potential/1 -> Sum3/2
  Constant10/1 -> Inertial Link With Reset1/2
  Synapses/1 -> Sum1/1
  Sum1/1 -> Gain3/1
  Constant12/1 -> Sum1/2
  Sum3/1 -> Inertial Link With Reset1/1  "Value"
  Inertial Link With Reset1/1 -> Out1/1
  Constant1/1 -> Inertial Link With Reset1/3
  Gain3/1 -> Sum3/1  "Input"
  Reset Signal/1 -> Inertial Link With Reset1/4

== system NeuroModelerLibrary/Sized Cells/Cell IaF 4x4/IaF Membrane Segment37 ==
  Synapses : Inport
  Resting Potential : Inport  Port=2
  Reset Signal : Inport  Port=3
  Constant1 : Constant  Value=V_reset
  Constant10 : Constant  Value=tau_m
  Constant12 : Constant  Value=I_const
  Gain3 : Gain  Gain=tau_m/Cm
  Inertial Link With Reset1 : $bdroot/Support/Inertial Link With Reset  SystemSampleTime=-1  VariantActivationTime=update diagram  Latency=0  AutoFrameSizeCalculation=off
  Sum1 : Sum
  Sum3 : Sum
  Out1 : Outport
  wires:
  Resting Potential/1 -> Sum3/2
  Constant10/1 -> Inertial Link With Reset1/2
  Synapses/1 -> Sum1/1
  Sum1/1 -> Gain3/1
  Constant12/1 -> Sum1/2
  Sum3/1 -> Inertial Link With Reset1/1  "Value"
  Inertial Link With Reset1/1 -> Out1/1
  Constant1/1 -> Inertial Link With Reset1/3
  Gain3/1 -> Sum3/1  "Input"
  Reset Signal/1 -> Inertial Link With Reset1/4

== system NeuroModelerLibrary/Sized Cells/Cell IaF 4x4/IaF Membrane Segment38 ==
  Synapses : Inport
  Resting Potential : Inport  Port=2
  Reset Signal : Inport  Port=3
  Constant1 : Constant  Value=V_reset
  Constant10 : Constant  Value=tau_m
  Constant12 : Constant  Value=I_const
  Gain3 : Gain  Gain=tau_m/Cm
  Inertial Link With Reset1 : $bdroot/Support/Inertial Link With Reset  SystemSampleTime=-1  VariantActivationTime=update diagram  Latency=0  AutoFrameSizeCalculation=off
  Sum1 : Sum
  Sum3 : Sum
  Out1 : Outport
  wires:
  Resting Potential/1 -> Sum3/2
  Constant10/1 -> Inertial Link With Reset1/2
  Synapses/1 -> Sum1/1
  Sum1/1 -> Gain3/1
  Constant12/1 -> Sum1/2
  Sum3/1 -> Inertial Link With Reset1/1  "Value"
  Inertial Link With Reset1/1 -> Out1/1
  Constant1/1 -> Inertial Link With Reset1/3
  Gain3/1 -> Sum3/1  "Input"
  Reset Signal/1 -> Inertial Link With Reset1/4

== system NeuroModelerLibrary/Sized Cells/Cell IaF 4x4/IaF Membrane Segment39 ==
  Synapses : Inport
  Resting Potential : Inport  Port=2
  Reset Signal : Inport  Port=3
  Constant1 : Constant  Value=V_reset
  Constant10 : Constant  Value=tau_m
  Constant12 : Constant  Value=I_const
  Gain3 : Gain  Gain=tau_m/Cm
  Inertial Link With Reset1 : $bdroot/Support/Inertial Link With Reset  SystemSampleTime=-1  VariantActivationTime=update diagram  Latency=0  AutoFrameSizeCalculation=off
  Sum1 : Sum
  Sum3 : Sum
  Out1 : Outport
  wires:
  Resting Potential/1 -> Sum3/2
  Constant10/1 -> Inertial Link With Reset1/2
  Synapses/1 -> Sum1/1
  Sum1/1 -> Gain3/1
  Constant12/1 -> Sum1/2
  Sum3/1 -> Inertial Link With Reset1/1  "Value"
  Inertial Link With Reset1/1 -> Out1/1
  Constant1/1 -> Inertial Link With Reset1/3
  Gain3/1 -> Sum3/1  "Input"
  Reset Signal/1 -> Inertial Link With Reset1/4
